simulink model "ADPLL_model"  (R2017a)
settings: Solver=VariableStepAuto  StartTime=0.0  StopTime=4e-4  FixedStep=1/(12*4*Fref)  RelTol=1e-3
values from neighbouring files (symbols this model uses):
  BBPFD_delay = 1e-12    [ADPLL_simulink.m]
  Ffree = Fref*N*0.95    (= 380000000)    [ADPLL_simulink.m]
  Fref = 25e6    (= 25000000)    [ADPLL_simulink.m]
  Kdco = 3e6    (= 3000000)    [ADPLL_simulink.m]
  Ki = 0.01    [ADPLL_simulink.m]
  Kp = 0.05    [ADPLL_simulink.m]
  N = 16    [ADPLL_simulink.m]
undefined symbols (not defined in the file): DCO_Noise, Ref_Noise
libraries: simulink_extras x3, simulink x2
settings Model: Creator=ECL328  LastModifiedBy=fransiskusyoga

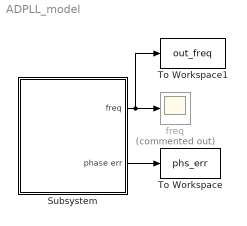
== system ADPLL_model ==
  Subsystem : Subsystem  mask{N=N, Kp=Kp, Ki=Ki, Kdco=Kdco, Fref=Fref, Ffree=Ffree, BBPFD_delay=BBPFD_delay, RefNoise=Ref_Noise, DCONoise=DCO_Noise}
      mask prompts: RefNoise "Var of RefNoise"; DCONoise "Var of DCONoise"
  To Workspace : ToWorkspace  VariableName=phs_err  SampleTime=-1
  To Workspace1 : ToWorkspace  VariableName=out_freq  SampleTime=-1
  freq : Scope  Commented=on
  wires:
  Subsystem/1(freq) -> To Workspace1/1, freq/1
  Subsystem/2(phase err) -> To Workspace/1

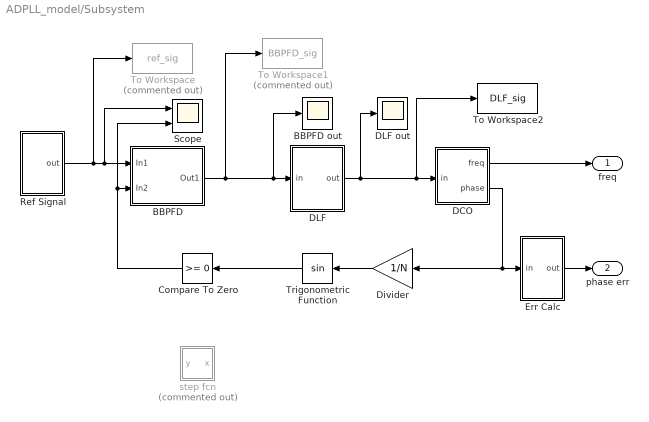
== system ADPLL_model/Subsystem ==
  BBPFD : Subsystem
  BBPFD out : Scope
  Compare To Zero : simulink/Logic and Bit Operations/Compare To Zero  relop=>=  OutDataTypeStr=boolean
  DCO : Subsystem
  DLF : Subsystem
  DLF out : Scope
  Divider : Gain  Gain=1/N
  Err Calc : Subsystem
  Ref Signal : Subsystem
  Scope : Scope  NumInputPorts=2
  To Workspace : ToWorkspace  Commented=on  VariableName=ref_sig  SaveFormat=Timeseries  SampleTime=-1
  To Workspace1 : ToWorkspace  Commented=on  VariableName=BBPFD_sig  SaveFormat=Timeseries  SampleTime=-1
  To Workspace2 : ToWorkspace  VariableName=DLF_sig  SampleTime=-1
  Trigonometric Function : Trigonometry
  step fcn : Subsystem  Commented=on
  freq : Outport
  phase err : Outport  Port=2
  wires:
  BBPFD/1(Out1) -> To Workspace1/1, BBPFD out/1, DLF/1(in)
  Divider/1 -> Trigonometric Function/1
  DLF/1(out) -> DLF out/1, To Workspace2/1, DCO/1(in)
  DCO/1(freq) -> freq/1
  Ref Signal/1(out) -> To Workspace/1, Scope/1, BBPFD/1(In1)
  Err Calc/1(out) -> phase err/1
  DCO/2(phase) -> Err Calc/1(in), Divider/1
  Trigonometric Function/1 -> Compare To Zero/1
  Compare To Zero/1 -> Scope/2, BBPFD/2(In2)

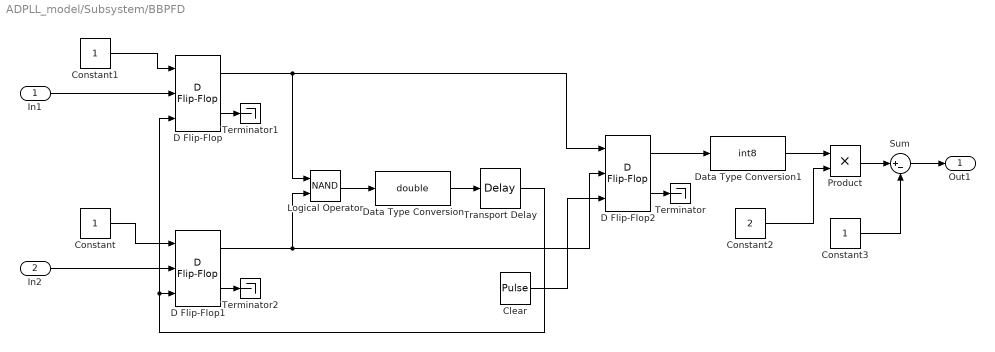
== system ADPLL_model/Subsystem/BBPFD ==
  In1 : Inport
  In2 : Inport  Port=2
  Clear : DiscretePulseGenerator  PulseType=Time based  Period=20  PulseWidth=50
  Constant : Constant  OutDataTypeStr=boolean
  Constant1 : Constant  OutDataTypeStr=boolean
  Constant2 : Constant  Value=2
  Constant3 : Constant
  D Flip-Flop : simulink_extras/Flip Flops/D Flip-Flop
      settings: SourceProductName=Simulink
  D Flip-Flop1 : simulink_extras/Flip Flops/D Flip-Flop
      settings: SourceProductName=Simulink
  D Flip-Flop2 : simulink_extras/Flip Flops/D Flip-Flop
      settings: SourceProductName=Simulink
  Data Type Conversion : DataTypeConversion  OutDataTypeStr=double
  Data Type Conversion1 : DataTypeConversion  OutDataTypeStr=int8
  Logical Operator : Logic  Operator=NAND  AllPortsSameDT=off  OutDataTypeStr=boolean
  Product : Product
  Sum : Sum  Inputs=|+-
  Terminator : Terminator
  Terminator1 : Terminator
  Terminator2 : Terminator
  Transport Delay : TransportDelay  DelayTime=BBPFD_delay
  Out1 : Outport
  wires:
  Data Type Conversion/1 -> Transport Delay/1
  Constant/1 -> D Flip-Flop1/1
  Sum/1 -> Out1/1
  D Flip-Flop2/1 -> Data Type Conversion1/1
  Product/1 -> Sum/1
  In1/1 -> D Flip-Flop/2
  Clear/1 -> D Flip-Flop2/3
  D Flip-Flop2/2 -> Terminator/1
  In2/1 -> D Flip-Flop1/2
  Constant3/1 -> Sum/2
  Data Type Conversion1/1 -> Product/1
  Constant1/1 -> D Flip-Flop/1
  Transport Delay/1 -> D Flip-Flop/3, D Flip-Flop1/3
  D Flip-Flop/1 -> D Flip-Flop2/1, Logical Operator/1
  D Flip-Flop1/1 -> Logical Operator/2, D Flip-Flop2/2
  Logical Operator/1 -> Data Type Conversion/1
  D Flip-Flop1/2 -> Terminator2/1
  Constant2/1 -> Product/2
  D Flip-Flop/2 -> Terminator1/1

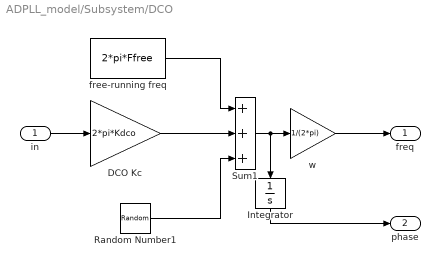
== system ADPLL_model/Subsystem/DCO ==
  in : Inport
  DCO Kc : Gain  Gain=2*pi*Kdco
  Integrator : Integrator
  Random Number1 : RandomNumber  Variance=DCONoise  SampleTime=1/(Fref*4)
  Sum1 : Sum  Inputs=+++
  free-running freq : Constant  Value=2*pi*Ffree
  w : Gain  Gain=1/(2*pi)
  freq : Outport
  phase : Outport  Port=2
  wires:
  in/1 -> DCO Kc/1
  Integrator/1 -> phase/1
  DCO Kc/1 -> Sum1/2
  Sum1/1 -> w/1, Integrator/1
  free-running freq/1 -> Sum1/1
  w/1 -> freq/1
  Random Number1/1 -> Sum1/3

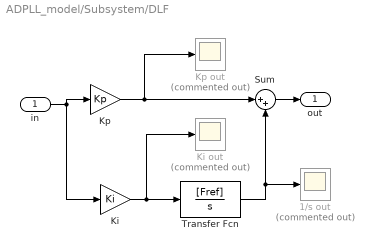
== system ADPLL_model/Subsystem/DLF ==
  in : Inport
  1/s out : Scope  Commented=on
  Ki : Gain  Gain=Ki
  Ki out : Scope  Commented=on
  Kp : Gain  Gain=Kp
  Kp out : Scope  Commented=on
  Sum : Sum  Inputs=|++
  Transfer Fcn : TransferFcn  Numerator=[Fref]  Denominator=[1 0]
  out : Outport
  wires:
  in/1 -> Kp/1, Ki/1
  Transfer Fcn/1 -> 1/s out/1, Sum/2
  Kp/1 -> Kp out/1, Sum/1
  Sum/1 -> out/1
  Ki/1 -> Ki out/1, Transfer Fcn/1

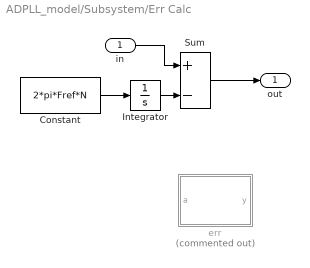
== system ADPLL_model/Subsystem/Err Calc ==
  in : Inport
  Constant : Constant  Value=2*pi*Fref*N
  Integrator : Integrator
  Sum : Sum  Inputs=+-
  err : MATLAB Function  Commented=on  TreatAsAtomicUnit=on
  out : Outport
  wires:
  Constant/1 -> Integrator/1
  Integrator/1 -> Sum/2
  in/1 -> Sum/1
  Sum/1 -> out/1

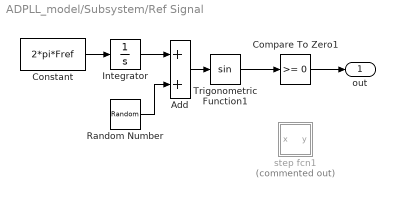
== system ADPLL_model/Subsystem/Ref Signal ==
  Add : Sum
  Compare To Zero1 : simulink/Logic and Bit Operations/Compare To Zero  relop=>=  OutDataTypeStr=boolean
  Constant : Constant  Value=2*pi*Fref
  Integrator : Integrator
  Random Number : RandomNumber  Variance=RefNoise  SampleTime=1/(4*Fref)
  Trigonometric Function1 : Trigonometry
  step fcn1 : Subsystem  Commented=on
  out : Outport
  wires:
  Random Number/1 -> Add/2
  Integrator/1 -> Add/1
  Add/1 -> Trigonometric Function1/1
  Trigonometric Function1/1 -> Compare To Zero1/1
  Compare To Zero1/1 -> out/1
  Constant/1 -> Integrator/1

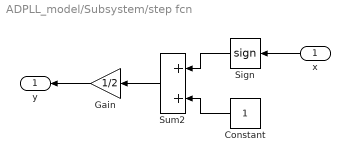
== system ADPLL_model/Subsystem/step fcn ==
  x : Inport
  Constant : Constant
  Gain : Gain  Gain=1/2
  Sign : Signum
  Sum2 : Sum
  y : Outport
  wires:
  Sum2/1 -> Gain/1
  Gain/1 -> y/1
  x/1 -> Sign/1
  Sign/1 -> Sum2/1
  Constant/1 -> Sum2/2

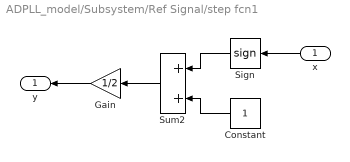
== system ADPLL_model/Subsystem/Ref Signal/step fcn1 ==
  x : Inport
  Constant : Constant
  Gain : Gain  Gain=1/2
  Sign : Signum
  Sum2 : Sum
  y : Outport
  wires:
  Sum2/1 -> Gain/1
  Gain/1 -> y/1
  x/1 -> Sign/1
  Sign/1 -> Sum2/1
  Constant/1 -> Sum2/2

== matlab function ADPLL_model/Subsystem/Err Calc/err ==
  data: a input; y output
function y = fcn(a)
temp = rem(a,2*pi);
y = temp - (2*pi)*(temp>pi);
